simulink library "Lib_Thermo_Enth2Temp_TMATS"  (R2019b)
settings: Solver=ode45  StartTime=0.0  StopTime=10.0  RelTol=1e-3  EnableMultiTasking=on
Description:
  | Thomas Modules
settings Model: Creator=jwchapm2  LastModifiedBy=bhisma
settings DataIOCC: LimitDataPoints=on  SaveFormat=Array  ReturnWorkspaceOutputs=off
settings OptimizationCC: ExpressionDepthLimit=2147483647  LifeSpan=inf
settings DebuggingCC: UnderspecifiedInitializationDetection=Classic  MergeDetectMultiDrivingBlocksExec=none  SolverPrmCheckMsg=warning  StateNameClashWarn=warning  SFUnexpectedBacktrackingDiag=warning  SFNoUnconditionalDefaultTransitionDiag=warning  SFExecutionAtInitializationDiag=none  ArithmeticOperatorsInVariantConditions=warning
settings HardwareCC: ProdBitPerPointer=32  ProdBitPerSizeT=32  ProdBitPerPtrDiffT=32  ProdLargestAtomicFloat=None  ProdIntDivRoundTo=Undefined  ProdEndianess=Unspecified  ProdWordSize=32  ProdHWDeviceType=32-bit Generic
settings ModelReferenceCC: PropagateSignalLabelsOutOfModel=off
settings SFSimCC: SimUseLocalCustomCode=off  CustomCodeUndefinedFunction=UseInterfaceOnly
settings RTWCC: RTWUseLocalCustomCode=off
settings CodeAppCC: StateflowObjectComments=on
settings GRTTargetCC: TargetLangStandard=C89/C90 (ANSI)  GeneratePreprocessorConditionals=Disable all
settings ConfigComp: CovMetricSettings=dw  CovHtmlReporting=on  CovSaveCumulativeToWorkspaceVar=on  CovSaveSingleToWorkspaceVar=on  CovExternalEMLEnable=off

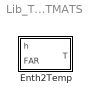
== system Lib_Thermo_Enth2Temp_TMATS ==
  Enth2Temp : Subsystem  mask(T-MATS: Enth2Temp Library Block){}
      mask help: This block emperically calculates temperature (T) from enthalpy (h) and fuel to air ratio (FAR).
      mask Help: web(which('Thermo_TMATS_Enth2Temp.html'),'-helpbrowser')

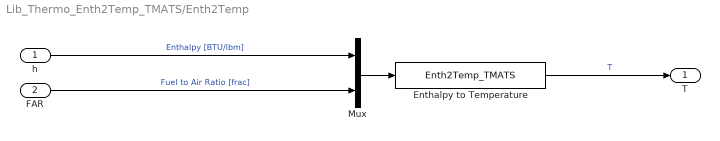
== system Lib_Thermo_Enth2Temp_TMATS/Enth2Temp ==
  h : Inport
  FAR : Inport  Port=2
  "Enthalpy to Temperature " : S-Function  FunctionName=Enth2Temp_TMATS  SFunctionModules='h2tc_TMATS'  SFunctionDeploymentMode=off  EnableBusSupport=off
  Mux : Mux  Inputs=2
  T : Outport
  wires:
  "Enthalpy to Temperature "/1 -> T/1  "T"
  Mux/1 -> "Enthalpy to Temperature "/1
  h/1 -> Mux/1  "Enthalpy [BTU/lbm]"
  FAR/1 -> Mux/2  "Fuel to Air Ratio [frac]"
